simulink model "divider"  (R2021a)
settings: Solver=VariableStepAuto  StartTime=0.0  StopTime=10.0  RelTol=1e-3
libraries: custom_lib x4
settings Model: Creator=Acer  LastModifiedBy=Acer

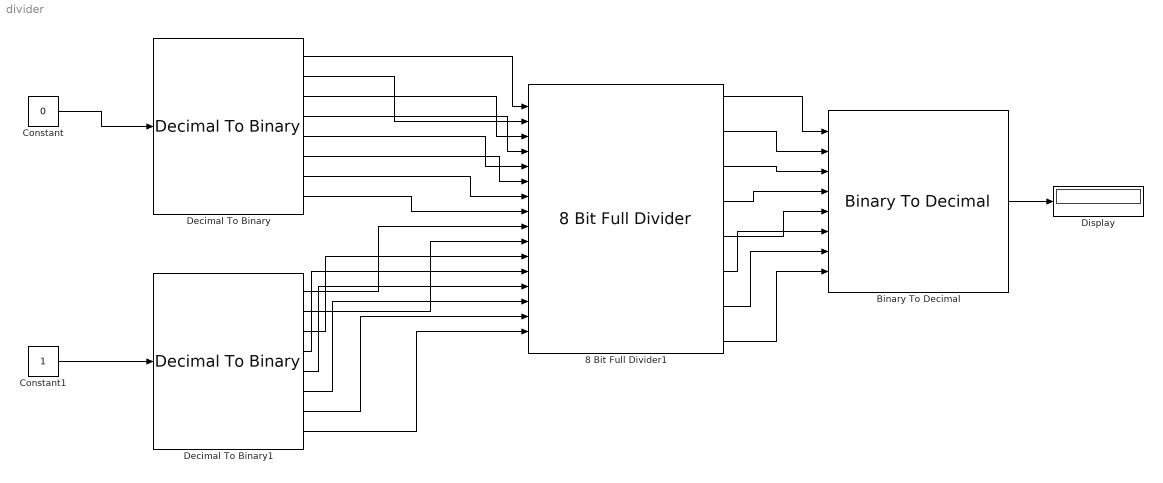
== system divider ==
  8 Bit Full Divider1 : custom_lib/8 Bit Full Divider  SystemSampleTime=-1  VariantActivationTime=update diagram  Latency=0  AutoFrameSizeCalculation=off
      settings: SourceProductName=Custom Library
  Binary To Decimal : custom_lib/Binary To Decimal  SystemSampleTime=-1  VariantActivationTime=update diagram  Latency=0  AutoFrameSizeCalculation=off
      settings: SourceProductName=Custom Library
  Constant : Constant  Value=0
  Constant1 : Constant
  Decimal To Binary : custom_lib/Decimal To Binary  SystemSampleTime=-1  VariantActivationTime=update diagram  Latency=0  AutoFrameSizeCalculation=off
      settings: SourceProductName=Custom Library
  Decimal To Binary1 : custom_lib/Decimal To Binary  SystemSampleTime=-1  VariantActivationTime=update diagram  Latency=0  AutoFrameSizeCalculation=off
      settings: SourceProductName=Custom Library
  Display : Display
  wires:
  Decimal To Binary/8 -> 8 Bit Full Divider1/8
  Decimal To Binary/7 -> 8 Bit Full Divider1/7
  Decimal To Binary/6 -> 8 Bit Full Divider1/6
  Decimal To Binary/5 -> 8 Bit Full Divider1/5
  Decimal To Binary/4 -> 8 Bit Full Divider1/4
  Decimal To Binary/3 -> 8 Bit Full Divider1/3
  Decimal To Binary/2 -> 8 Bit Full Divider1/2
  Decimal To Binary/1 -> 8 Bit Full Divider1/1
  Decimal To Binary1/8 -> 8 Bit Full Divider1/16
  Decimal To Binary1/7 -> 8 Bit Full Divider1/15
  Decimal To Binary1/6 -> 8 Bit Full Divider1/14
  Decimal To Binary1/5 -> 8 Bit Full Divider1/13
  Decimal To Binary1/4 -> 8 Bit Full Divider1/12
  Decimal To Binary1/3 -> 8 Bit Full Divider1/11
  Decimal To Binary1/2 -> 8 Bit Full Divider1/10
  Decimal To Binary1/1 -> 8 Bit Full Divider1/9
  8 Bit Full Divider1/8 -> Binary To Decimal/8
  8 Bit Full Divider1/7 -> Binary To Decimal/7
  8 Bit Full Divider1/6 -> Binary To Decimal/6
  8 Bit Full Divider1/5 -> Binary To Decimal/5
  8 Bit Full Divider1/4 -> Binary To Decimal/4
  8 Bit Full Divider1/3 -> Binary To Decimal/3
  8 Bit Full Divider1/2 -> Binary To Decimal/2
  8 Bit Full Divider1/1 -> Binary To Decimal/1
  Binary To Decimal/1 -> Display/1
  Constant/1 -> Decimal To Binary/1
  Constant1/1 -> Decimal To Binary1/1
